simulink library "GOcontroll_Crank"  (R2023b)
settings: Solver=ode45  StartTime=0.0  StopTime=10.0  RelTol=1e-3  EnableMultiTasking=on
PreLoadFcn:
  | compile_crank_mex;
undefined symbols (not defined in the file or in its folder): DiscIntNeverNeededParam, missing
libraries: simulink x2
(part 2 of 2)

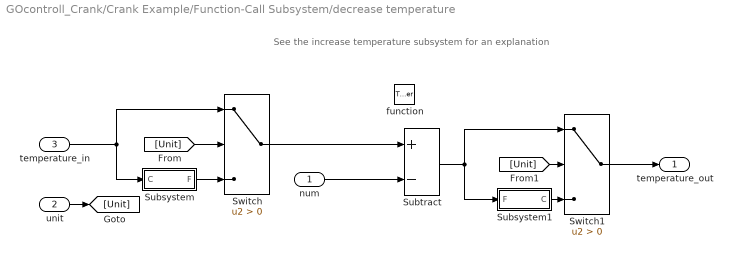
== system GOcontroll_Crank/Crank Example/Function-Call Subsystem/decrease temperature ==
  note: See the increase temperature subsystem for an explanation
  num : Inport
  unit : Inport  Port=2
  temperature_in : Inport  Port=3  Unit=degC
  function : TriggerPort  TriggerType=function-call  VariantControl=(inherit)
  Subsystem : Subsystem
  Subsystem1 : Subsystem
  Subtract : Sum  Inputs=+-  OutDataTypeStr=single  AccumDataTypeStr=single
  Switch : Switch  Criteria=u2 > Threshold  SaturateOnIntegerOverflow=off  InputSameDT=off
  Switch1 : Switch  Criteria=u2 > Threshold  SaturateOnIntegerOverflow=off  InputSameDT=off
  temperature_out : Outport  InitialOutput=int16(16)
  wires:
  Subsystem1/1(C) -> Switch1/3
  Subsystem/1(F) -> Switch/3
  Switch1/1 -> temperature_out/1
  [Unit] -> Switch1/2
  Switch/1 -> Subtract/1
  [Unit] -> Switch/2
  unit/1 -> [Unit]
  Subtract/1 -> Switch1/1, Subsystem1/1(F)
  temperature_in/1 -> Switch/1, Subsystem/1(C)
  num/1 -> Subtract/2

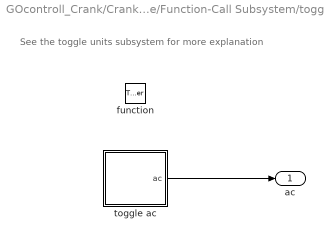
== system GOcontroll_Crank/Crank Example/Function-Call Subsystem/toggle ac ==
  note: See the toggle units subsystem for more explanation
  function : TriggerPort  TriggerType=function-call  VariantControl=(inherit)
  toggle ac : Stateflow chart  TreatAsAtomicUnit=on
  ac : Outport
  wires:
  toggle ac/1(ac) -> ac/1

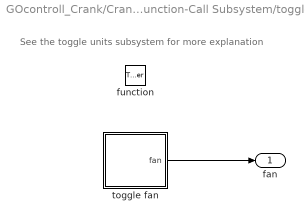
== system GOcontroll_Crank/Crank Example/Function-Call Subsystem/toggle fan ==
  note: See the toggle units subsystem for more explanation
  function : TriggerPort  TriggerType=function-call  VariantControl=(inherit)
  toggle fan : Stateflow chart  TreatAsAtomicUnit=on
  fan : Outport
  wires:
  toggle fan/1(fan) -> fan/1

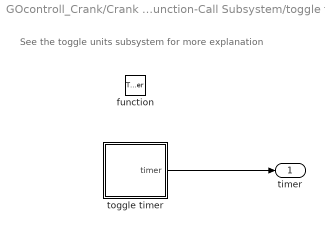
== system GOcontroll_Crank/Crank Example/Function-Call Subsystem/toggle timer ==
  note: See the toggle units subsystem for more explanation
  function : TriggerPort  TriggerType=function-call  VariantControl=(inherit)
  toggle timer : Stateflow chart  TreatAsAtomicUnit=on
  timer : Outport
  wires:
  toggle timer/1(timer) -> timer/1

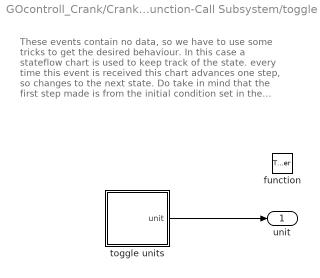
== system GOcontroll_Crank/Crank Example/Function-Call Subsystem/toggle units ==
  note: These events contain no data, so we have
      | to use some tricks to get the desired
      | behaviour.
      | In this case a stateflow chart is used to
      | keep track of the state. every time this
      | event is received this chart advances one
      | step, so changes to the next state.
      | Do take in mind that the first step made is
      | from the initial condition set in the 'explore'
      | window to the first actual state.
  function : TriggerPort  TriggerType=function-call  VariantControl=(inherit)
  toggle units : Stateflow chart  TreatAsAtomicUnit=on
  unit : Outport
  wires:
  toggle units/1(unit) -> unit/1

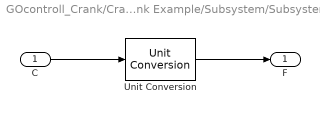
== system GOcontroll_Crank/Crank Example/Subsystem/Subsystem ==
  C : Inport  Unit=degC
  Unit Conversion : UnitConversion  OutputType=Inherit: Inherit via back propagation
  F : Outport  OutDataTypeStr=int16  Unit=degF
  wires:
  Unit Conversion/1 -> F/1
  C/1 -> Unit Conversion/1

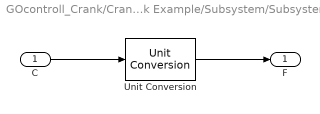
== system GOcontroll_Crank/Crank Example/Subsystem/Subsystem1 ==
  C : Inport  Unit=degC
  Unit Conversion : UnitConversion  OutputType=Inherit: Inherit via back propagation
  F : Outport  OutDataTypeStr=int16  Unit=degF
  wires:
  C/1 -> Unit Conversion/1
  Unit Conversion/1 -> F/1

== system GOcontroll_Crank/Crank Example/Function-Call Subsystem/Increase temperature/Subsystem ==
  C : Inport  Unit=degC
  Unit Conversion : UnitConversion  OutputType=Inherit: Inherit via back propagation
  F : Outport  OutDataTypeStr=single  Unit=degF
  wires:
  Unit Conversion/1 -> F/1
  C/1 -> Unit Conversion/1

== system GOcontroll_Crank/Crank Example/Function-Call Subsystem/Increase temperature/Subsystem1 ==
  F : Inport  Unit=degF
  Unit Conversion : UnitConversion  OutputType=Inherit: Inherit via back propagation
  C : Outport  OutDataTypeStr=single  Unit=degC
  wires:
  F/1 -> Unit Conversion/1
  Unit Conversion/1 -> C/1

== system GOcontroll_Crank/Crank Example/Function-Call Subsystem/decrease temperature/Subsystem ==
  C : Inport  Unit=degC
  Unit Conversion : UnitConversion  OutputType=Inherit: Inherit via back propagation
  F : Outport  OutDataTypeStr=single  Unit=degF
  wires:
  Unit Conversion/1 -> F/1
  C/1 -> Unit Conversion/1

== system GOcontroll_Crank/Crank Example/Function-Call Subsystem/decrease temperature/Subsystem1 ==
  F : Inport  Unit=degF
  Unit Conversion : UnitConversion  OutputType=Inherit: Inherit via back propagation
  C : Outport  OutDataTypeStr=single  Unit=degC
  wires:
  F/1 -> Unit Conversion/1
  Unit Conversion/1 -> C/1

== stateflow chart GOcontroll_Crank/Crank Example/Function-Call Subsystem/toggle ac/toggle ac ==
  note: The initial value of ac is set to 0 in the 'explore' window
      | If it is not done this way, it takes to presses to switch the
      | first time.
  state on
    en: ac = 1;
  state off
    en: ac = 0;
  (default) -> on
  on -> off
  off -> on
  data: ac output uint8 =uint8(0)

== stateflow chart GOcontroll_Crank/Crank Example/Function-Call Subsystem/toggle units/toggle units ==
  note: The initial value of unit is set to 1 in the 'explore' window
      | If it is not done this way, it takes to presses to switch the
      | first time.
  state fahrenheit
    en: unit = 0;
  state celsius
    en: unit = 1;
  (default) -> fahrenheit
  fahrenheit -> celsius
  celsius -> fahrenheit
  data: unit output uint8 =uint8(1)
  data unit settings: description=In the example the default state of unit is 1 which equals celsius, so the initialValue here has to be 1

== stateflow chart GOcontroll_Crank/Crank Example/Function-Call Subsystem/toggle fan/toggle fan ==
  note: The initial value of fan is set to 0 in the 'explore' window
      | If it is not done this way, it takes to presses to switch the
      | first time.
  state on
    en: fan = 1;
  state off
    en: fan = 0;
  (default) -> on
  on -> off
  off -> on
  data: fan output uint8 =uint8(0)

== stateflow chart GOcontroll_Crank/Crank Example/Function-Call Subsystem/toggle timer/toggle timer ==
  note: The initial value of timer is set to 0 in the 'explore' window
      | If it is not done this way, it takes to presses to switch the
      | first time.
  state on
    en: timer = 1;
  state off
    en: timer = 0;
  (default) -> on
  on -> off
  off -> on
  data: timer output uint8 =uint8(0)
